simulink model "PMSM_FOC_CompVer"  (R2017b)
settings: Solver=FixedStepAuto  StartTime=0.0  StopTime=10.0  FixedStep=1e-6  RelTol=1e-3  AbsTol=1e-3
model workspace (MAT data in the model file):
  Ts = Simulink.Parameter
  Ts.Value = 0.001
  Ts.DataType = 'auto'
  Ts.Dimensions = [1 1]
libraries: nesl_utility x13, fl_lib x9, ee_lib x5, powerlib x4, simulink x3, powerlib_meascontrol x3, eeTransforms x2
settings Model: Creator=ljz  LastModifiedBy=ljz
settings DataIOCC: ReturnWorkspaceOutputs=on
settings DebuggingCC: SymbolicDimsDataTypeCodeGenerationDiagnostic=none
settings SFSimCC: SimUseLocalCustomCode=on
settings RTWCC: RTWUseLocalCustomCode=on
settings SimscapeCC: SimscapeLogType=all  SimscapeLogSimulationStatistics=on  SimscapeLogDataHistory=10000

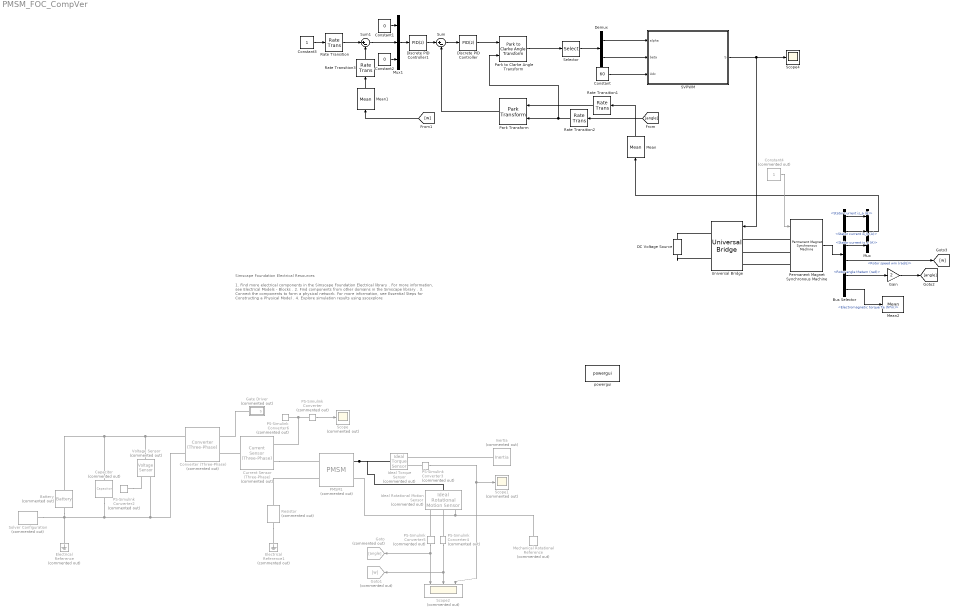
== system PMSM_FOC_CompVer ==
  note: 1. Find more electrical components in the Simscape Foundation Electrical library .
      | For more information, see Electrical Models - Blocks .
      | 2. Find components from other domains in the Simscape library .
      | 3. Connect the components to form a physical network.
      | For more information, see Essential Steps for Constructing a Physical Model .
      | 4. Explore simulation results using sscexplore
  note: Simscape Foundation Electrical Resources
  Battery : ee_lib/Sources/Battery  Commented=on  Vnom=12 V  R1=2 Ohm  prm_AH=1  AH=50 hr*A  V1=11.5 V  AH1=25 hr*A  prm_R2=1  R2=2000 Ohm  prm_dyn=1  Rp1=0.005 Ohm  tau1=30 s  Rp2=0.005 Ohm  tau2=30 s  Rp3=0.005 Ohm  tau3=30 s  Rp4=0.005 Ohm  tau4=30 s  Rp5=0.005 Ohm  tau5=30 s  prm_fade=1  N_fade=100  AH_fade=45 hr*A  R1_fade=2.02 Ohm  V1_fade=10.35 V  i_specify=off  i_priority=None  i=0 A  i_nominal_specify=off  i_nominal_unit=A  i_nominal_value=1  v_specify=off  v_priority=None  v=0 V  v_nominal_specify=off  v_nominal_unit=V  v_nominal_value=1  charge_specify=off  charge_priority=High  charge=50 hr*A  charge_nominal_specify=off  charge_nominal_unit=hr*A  charge_nominal_value=1  num_cycles_specify=off  num_cycles_priority=High  num_cycles=0  num_cycles_nominal_specify=off  num_cycles_nominal_unit=1  num_cycles_nominal_value=1  thermal_mass=30000 J/K  Tmeas=298.15 K  Vnom_T2=12 V  R1_T2=2.2 Ohm  V1_T2=11.4 V  R2_T2=2200 Ohm  Rp1_T2=0.005 Ohm  tau1_T2=30 s  Rp2_T2=0.005 Ohm  tau2_T2=30 s  Rp3_T2=0.005 Ohm  tau3_T2=30 s  Rp4_T2=0.005 Ohm  tau4_T2=30 s  Rp5_T2=0.005 Ohm  tau5_T2=30 s  Tmeas2=273.15 K  temperature_specify=off  temperature_priority=High  temperature=298.15 K  temperature_nominal_specify=off  temperature_nominal_unit=K  temperature_nominal_value=1
  Bus Selector : BusSelector  OutputSignals=Stator current is_a (A),Stator current is_b (A),Stator current is_c (A),Rotor speed wm (rad/s),Rotor angle thetam (rad),Electromagnetic torque Te (N*m)
  Capacitor : fl_lib/Electrical/Electrical Elements/Capacitor  Commented=on  c=220 uF  r=1e-6 Ohm  g=0 1/Ohm  i_specify=off  i_priority=None  i=0 A  i_nominal_specify=off  i_nominal_unit=A  i_nominal_value=1  v_specify=off  v_priority=None  v=0 V  v_nominal_specify=off  v_nominal_unit=V  v_nominal_value=1  vc_specify=off  vc_priority=High  vc=0 V  vc_nominal_specify=off  vc_nominal_unit=V  vc_nominal_value=1
  Constant : Constant  Value=60
  Constant1 : Constant  Value=0
  Constant2 : Constant  Value=0
  Constant3 : Constant
  Constant4 : Constant  Commented=on
  Converter (Three-Phase) : ee_lib/Semiconductors & Converters/Converters/Converter (Three-Phase)  Commented=on  device_type=ee.enum.converters.switchingdevice.ideal  Vf=0.8 V  Ron=0.001 Ohm  Rds=0.001 Ohm  Goff=1e-6 1/Ohm  Vth=0.5 V  Vgt=1 V  Vgt_off=-1 V  Ih=1 A  diode_param=ee.enum.converters.protectiondiode.none  diode_Vf=0.8 V  diode_Ron=0.001 Ohm  diode_Goff=1e-5 1/Ohm  diode_C=50 nF  diode_iRM=-235 A  diode_iF=300 A  diode_idot=-50 A/us  diode_trr_param=ee.enum.converters.diodetrr.trr_factor  diode_trr_factor=3  diode_trr=15 us  diode_Qrr=1500 s*uA  snubber_type=ee.enum.converters.snubber.exclude  Rs=0.1 Ohm  Cs=1e-7 F
      settings: SourceProductBaseCode=PS
  Current Sensor (Three-Phase) : ee_lib/Sensors & Transducers/Current Sensor (Three-Phase)  Commented=on
  DC Voltage Source : powerlib/Electrical Sources/DC Voltage Source  Amplitude=60  Measurements=None
  Demux : Demux  Outputs=2
  Discrete PID Controller : simulink/Continuous/PID Controller  Controller=PID  Form=Parallel  TimeDomain=Discrete-time  SampleTime=-1  IntegratorMethod=Forward Euler  FilterMethod=Forward Euler  ControllerParametersSource=internal  P=10  I=10  D=0  UseFilter=on  N=100  TunerSelectOption=Transfer Function Based (PID Tuner App)  InitialConditionSource=internal  InitialConditionForIntegrator=0  InitialConditionForFilter=0  DifferentiatorICPrevScaledInput=0  ExternalReset=none  TrackingMode=off  Kt=1  LimitOutput=off  UpperSaturationLimit=inf  LowerSaturationLimit=-inf  LinearizeAsGain=off  AntiWindupMode=none  Kb=1  POutMin=[]  POutMax=[]  IOutMin=[]  IOutMax=[]  DOutMin=[]  DOutMax=[]  NOutMin=[]  NOutMax=[]  SumOutMin=[]  SumOutMax=[]  SaturationOutMin=[]  SaturationOutMax=[]  PParamMin=[]  PParamMax=[]  IParamMin=[]  IParamMax=[]  DParamMin=[]  DParamMax=[]  NParamMin=[]  NParamMax=[]  KbParamMin=[]  KbParamMax=[]  KtParamMin=[]  KtParamMax=[]  KbOutMin=[]  KbOutMax=[]  KtOutMin=[]  KtOutMax=[]  IntegratorOutMin=[]  IntegratorOutMax=[]  FilterOutMin=[]  FilterOutMax=[]  SumI1OutMin=[]  SumI1OutMax=[]  SumI2OutMin=[]  SumI2OutMax=[]  SumI3OutMin=[]  SumI3OutMax=[]  SumDOutMin=[]  SumDOutMax=[]  DifferentiatorOutMin=[]  DifferentiatorOutMax=[]  FilterDiffOutCoefMin=[]  FilterDiffOutCoefMax=[]  ReciprocalOutMin=[]  ReciprocalOutMax=[]  SumDenOutMin=[]  SumDenOutMax=[]  SumNumOutMin=[]  SumNumOutMax=[]  DivideOutMin=[]  DivideOutMax=[]  IntegratorContinuousStateAttributes=''  IntegratorStateMustResolveToSignalObject=off  IntegratorRTWStateStorageClass=Auto  FilterContinuousStateAttributes=''  FilterStateMustResolveToSignalObject=off  FilterRTWStateStorageClass=Auto
  Discrete PID Controller1 : simulink/Continuous/PID Controller  Controller=PID  Form=Parallel  TimeDomain=Discrete-time  SampleTime=-1  IntegratorMethod=Forward Euler  FilterMethod=Forward Euler  ControllerParametersSource=internal  P=0.06  I=1  D=0  UseFilter=on  N=100  TunerSelectOption=Transfer Function Based (PID Tuner App)  InitialConditionSource=internal  InitialConditionForIntegrator=0  InitialConditionForFilter=0  DifferentiatorICPrevScaledInput=0  ExternalReset=none  TrackingMode=off  Kt=1  LimitOutput=off  UpperSaturationLimit=inf  LowerSaturationLimit=-inf  LinearizeAsGain=off  AntiWindupMode=none  Kb=1  POutMin=[]  POutMax=[]  IOutMin=[]  IOutMax=[]  DOutMin=[]  DOutMax=[]  NOutMin=[]  NOutMax=[]  SumOutMin=[]  SumOutMax=[]  SaturationOutMin=[]  SaturationOutMax=[]  PParamMin=[]  PParamMax=[]  IParamMin=[]  IParamMax=[]  DParamMin=[]  DParamMax=[]  NParamMin=[]  NParamMax=[]  KbParamMin=[]  KbParamMax=[]  KtParamMin=[]  KtParamMax=[]  KbOutMin=[]  KbOutMax=[]  KtOutMin=[]  KtOutMax=[]  IntegratorOutMin=[]  IntegratorOutMax=[]  FilterOutMin=[]  FilterOutMax=[]  SumI1OutMin=[]  SumI1OutMax=[]  SumI2OutMin=[]  SumI2OutMax=[]  SumI3OutMin=[]  SumI3OutMax=[]  SumDOutMin=[]  SumDOutMax=[]  DifferentiatorOutMin=[]  DifferentiatorOutMax=[]  FilterDiffOutCoefMin=[]  FilterDiffOutCoefMax=[]  ReciprocalOutMin=[]  ReciprocalOutMax=[]  SumDenOutMin=[]  SumDenOutMax=[]  SumNumOutMin=[]  SumNumOutMax=[]  DivideOutMin=[]  DivideOutMax=[]  IntegratorContinuousStateAttributes=''  IntegratorStateMustResolveToSignalObject=off  IntegratorRTWStateStorageClass=Auto  FilterContinuousStateAttributes=''  FilterStateMustResolveToSignalObject=off  FilterRTWStateStorageClass=Auto
  Electrical Reference : fl_lib/Electrical/Electrical Elements/Electrical Reference  Commented=on
  Electrical Reference1 : fl_lib/Electrical/Electrical Elements/Electrical Reference  Commented=on
  Gain : Gain  Gain=2
  Gate Driver : Subsystem  Commented=on
  Goto : Goto  Commented=on  GotoTag=angle
  Goto1 : Goto  Commented=on  GotoTag=w
  Ideal Rotational Motion Sensor : fl_lib/Mechanical/Mechanical Sensors/Ideal Rotational Motion Sensor  Commented=on  wrap_angle=simscape.enum.onoff.off  offset=0 rad
  Ideal Torque Sensor : fl_lib/Mechanical/Mechanical Sensors/Ideal Torque Sensor  Commented=on
  Inertia : fl_lib/Mechanical/Rotational Elements/Inertia  Commented=on  inertia=0.01 kg*m^2  w_specify=off  w_priority=High  w=0 rad/s  w_nominal_specify=off  w_nominal_unit=rad/s  w_nominal_value=1  t_specify=off  t_priority=None  t=0 N*m  t_nominal_specify=off  t_nominal_unit=N*m  t_nominal_value=1
  Mean : powerlib_meascontrol/Measurements/Mean  Freq=1000  Vinit=0  Ts=0
  Mean1 : powerlib_meascontrol/Measurements/Mean  Freq=1000  Vinit=0  Ts=0
  Mean2 : powerlib_meascontrol/Measurements/Mean  Freq=1000  Vinit=0  Ts=0
  Mechanical Rotational Reference : fl_lib/Mechanical/Rotational Elements/Mechanical Rotational Reference  Commented=on
  Mux : Mux  Inputs=3
  Mux1 : Mux  Inputs=3
  PMSM1 : ee_lib/Electromechanical/Permanent Magnet/PMSM  Commented=on  winding_type=ee.enum.statorconnection.wye  machine_param=ee.enum.pmsm.parameterization.constant  nPolePairs=6  pmflux_param=ee.enum.pmflux.fluxlinkage  pm_flux_linkage=0.03 Wb  torque_constant=0.18 N*m/A  back_emf_constant=0.18 V/(rad/s)  stator_param=ee.enum.statorparam.LdLqL0  Ld=0.00019 H  Lq=0.00025 H  idVec=[-200, 0, 200] A  iqVec=[-200, 0, 200] A  LdMatrix=0.0002 * ones(3, 3) H  LqMatrix=0.0002 * ones(3, 3) H  PmMatrix=0.1 * ones(3, 3) Wb  ktMatrix=0.18 * ones(3, 3) N*m/A  keMatrix=0.18 * ones(3, 3) V/(rad/s)  L0=0.00016 H  Ls=0.0002 H  Lm=-0.00002 H  Ms=0.00002 H  Rs=0.013 Ohm  zero_sequence=ee.enum.park.zerosequence.include  J=0.01 kg*m^2  lam=0 N*m/(rad/s)  axes_param=ee.enum.rotorangle.daxis  i_d_specify=off  i_d_priority=None  i_d=0 A  i_d_nominal_specify=off  i_d_nominal_unit=A  i_d_nominal_value=1  i_q_specify=off  i_q_priority=None  i_q=0 A  i_q_nominal_specify=off  i_q_nominal_unit=A  i_q_nominal_value=1  torque_specify=off  torque_priority=None  torque=0 N*m  torque_nominal_specify=off  torque_nominal_unit=N*m  torque_nominal_value=1  angular_velocity_specify=off  angular_velocity_priority=High  angular_velocity=0 rpm  angular_velocity_nominal_specify=off  angular_velocity_nominal_unit=rpm  angular_velocity_nominal_value=1  angular_position_specify=off  angular_position_priority=High  angular_position=0 deg  angular_position_nominal_specify=off  angular_position_nominal_unit=deg  angular_position_nominal_value=1  loss_param=ee.enum.ironloss.none  losses_oc=[0, 0, 0] W  losses_sc=[0, 0, 0] W  f_losses=60 Hz  Isc_losses=95 A  Tmeas=298.15 K  alpha=3.93e-3 1/K  alpha_flux=-0.001 1/K  stator_thermal_mass=100 J/K  rotor_thermal_mass=200 J/K  Rm_percent_rotor=90  Rd_percent_rotor=30  temperatureA_specify=off  temperatureA_priority=High  temperatureA=25 degC  temperatureA_nominal_specify=off  temperatureA_nominal_unit=degC  temperatureA_nominal_value=1  temperatureB_specify=off  temperatureB_priority=High  temperatureB=25 degC  temperatureB_nominal_specify=off  temperatureB_nominal_unit=degC  temperatureB_nominal_value=1  temperatureC_specify=off  temperatureC_priority=High  temperatureC=25 degC  temperatureC_nominal_specify=off  temperatureC_nominal_unit=degC  temperatureC_nominal_value=1  temperatureR_specify=off  temperatureR_priority=High  temperatureR=25 degC  temperatureR_nominal_specify=off  temperatureR_nominal_unit=degC  temperatureR_nominal_value=1
      settings: InternalSimscapePortConfiguration="{\"Bottom\":[],\"Left\":[{\"id\":\"N\",\"label\":\"~\",\"type\":\"foundation.electrical.three_phase\"},{\"id\":\"n\",\"label\":\"n\",\"type\":\"foundation.electrical.electrical\"}],\"Right\":[{\"id\":\"R\",\"label\":\"R\",\"type\":\"foundation.mechanical.rotational.rotational\"},{\"id\":\"C\",\"label\":\"C\",\"type\":\"foundation.mechanical.rotational.rotational\"}],\"Top\":[]}"
  PS-Simulink Converter{,2..6} (6 alike) : nesl_utility/PS-Simulink Converter  Commented=on  PhysicalDomain=network_engine_domain  SubClassName=ps_output  LeftPortType=input  RightPortType=output  PseudoPeriodic=off  Frequencies=[]  Unit=inherit  AffineConversion=off
  Park Transform : eeTransforms/Park Transform  AxisAlignment=D-axis  PowerInvariant=off
  Park to Clarke Angle Transform : eeTransforms/Park to Clarke Angle Transform  AxisAlignment=D-axis
      settings: SourceProductBaseCode=PS
  Permanent Magnet Synchronous Machine : powerlib/Machines/Permanent Magnet Synchronous Machine  NbPhases=3  FluxDistribution=Sinusoidal  RotorType=Round  MechanicalLoad=Torque Tm  PresetModel=No  ShowDetailedParameters=on  MeasurementBus=off  Resistance=18.7  Inductance=8.5e-3  dqInductances=[8.5e-3,8.5e-3]  La=0.02682  MachineConstant=Flux linkage established by magnets (V.s)  Flux=0.1716  VoltageCst=62.2496  TorqueCst=0.5148  Flat=120  Mechanical=[2.26e-05 1.349e-05 2 0]  PolePairs=2  InitialConditions=[0,0, 0,0]  InitialConditions5ph=[0 0 0 0 0 0]  RefAngle=Aligned with phase A axis (original Park)  IterativeDiscreteModel=Trapezoidal non iterative  TsBlock=-1  TsPowergui=0
  Rate Transition{,1..3} (4 alike) : RateTransition  OutPortSampleTime=0.001
  Resistor : fl_lib/Electrical/Electrical Elements/Resistor  Commented=on  R=100 Ohm  i_specify=off  i_priority=None  i=0 A  i_nominal_specify=off  i_nominal_unit=A  i_nominal_value=1  v_specify=off  v_priority=None  v=0 V  v_nominal_specify=off  v_nominal_unit=V  v_nominal_value=1
  SVPWM : Subsystem
  Scope : Scope  Commented=on
  Scope1 : Scope  Commented=on
  Scope2 : Scope  Commented=on  NumInputPorts=3
  Scope4 : Scope
  Selector : Selector  InputPortWidth=3  IndexOptions=Index vector (dialog)  Indices=[1 2]  OutputSizes=1
  Solver Configuration : nesl_utility/Solver Configuration  Commented=on  PhysicalDomain=network_engine_domain  SubClassName=solver  LeftPortType=input  RightPortType=generic  Tones=[]  Harmonics=[]  SimulateNoise=off  Profile=off  UseLocalSampling=off  EnableSwitchedLinearOptims=on  FrequencyDomain=off  UseCCode=off  RelTol=0.001  AbsTol=1e-06  MinStep=1e-09  ToWorkspace=off  RevertToSquareIcSolve=off  NumHomotopyIterations=100  PhasorMode=off  PhasorModeNumHarmonics=1  DoDC=off  ResidualTolerance=1e-09  UseLocalSolver=off  LocalSolverChoice=NE_BACKWARD_EULER_ADVANCER  LocalSolverSampleTime=0.001  DoFixedCost=off  MaxNonlinIter=3  MaxModeIter=2  LinearAlgebra=auto  EquationFormulation=NE_TIME_EF  DelaysMemoryBudget=1024  AutomaticFiltering=on  FilteringTimeConstant=0.001  PartitionStorageMethod=AS_NEEDED  PartitionMemoryBudget=1024  PartitionMethod=ROBUST
  Sum : Sum  Inputs=|+-
  Sum1 : Sum  Inputs=|+-
  Universal Bridge : powerlib/Power Electronics/Universal Bridge  Arms=3  SnubberResistance=1e5  SnubberCapacitance=inf  Device=IGBT / Diodes  Ron=1e-3  Lon=0  ForwardVoltages="[  0  0  ]"  ForwardVoltage=0  GTOparameters=[ 10e-6 , 20e-6 ]  IGBTparameters=[ 1e-6 , 2e-6 ]  Measurements=None  Measurements_2=None  converterType=Rectifier
  Voltage Sensor : fl_lib/Electrical/Electrical Sensors/Voltage Sensor  Commented=on
  powergui : powerlib/powergui  Priority=1  SimulationMode=Discrete  SampleTime=1e-6  frequency=60  Iterations=50  frequencyindice=0  Pbase=100e6  ErrMax=1e-4  UnitsV=kV  UnitsW=MW  buscounter=0  FunctionMessages=off  echomessages=off  EnableUseOfTLC=off  CurrentSourceSwitches=off  DisableSnubberDevices=off  DisableRonSwitches=off  DisableVfSwitches=off  DisplayEquations=off  AutomaticDiscreteSolvers=off  SolverType=Tustin/Backward Euler (TBE)  Interpol=off  ExternalGateDelay=off  methode=off  Ts=100  x0status=blocks  SPID=on  SwTol=0  HookPort=off  NonlinearTolerance=1e-4  nMaxIteration=100  ContinueOnMaxIteration=off  RestoreLinks=warning  ResistiveCurrentMeasurement=off  Frange=[0:2:500]  Ylog=off  Xlog=on  ShowGrid=off  save=off  variable=ZData  structure=0  ZoomFFT=off  StartTime=0.0  cycles=1  DisplayStyle=1  fundamental=60  FreqAxis=off  MaxFrequency=1000  frequencyindicesteady=1  RmsSteady=1  display=off
  wires:
  PS-Simulink Converter4/1 -> Goto1/1, Scope2/2
  PS-Simulink Converter3/1 -> Scope2/3, Scope1/1
  PS-Simulink Converter5/1 -> Scope2/1, Goto/1
  PS-Simulink Converter/1 -> Scope/1
  [angle] -> Rate Transition2/1
  Selector/1 -> Demux/1
  Park to Clarke Angle Transform/1 -> Selector/1
  Sum/1 -> Discrete PID Controller/1
  Discrete PID Controller/1 -> Park to Clarke Angle Transform/1
  Constant3/1 -> Rate Transition/1
  Rate Transition1/1 -> Park Transform/1
  Rate Transition2/1 -> Park to Clarke Angle Transform/2, Park Transform/2
  Permanent Magnet Synchronous Machine/1 -> Bus Selector/1
  Bus Selector/1 -> Mux/1  "<Stator current is_a (A)>"
  Bus Selector/2 -> Mux/2  "<Stator current is_b (A)>"
  Bus Selector/3 -> Mux/3  "<Stator current is_c (A)>"
  Mux/1 -> Mean/1
  Bus Selector/4 -> [w]  "<Rotor speed wm (rad/s)>"
  Bus Selector/5 -> Gain/1  "<Rotor angle thetam (rad)>"
  Park Transform/1 -> Sum/2
  Mean/1 -> Rate Transition1/1
  Gain/1 -> [angle]
  Demux/1 -> SVPWM/1(alpha)
  Demux/2 -> SVPWM/2(beta)
  Constant/1 -> SVPWM/3(Udc)
  SVPWM/1(S) -> Scope4/1, Universal Bridge/1
  Discrete PID Controller1/1 -> Sum/1
  [w] -> Mean1/1
  Mean1/1 -> Rate Transition3/1
  Rate Transition3/1 -> Sum1/2
  Rate Transition/1 -> Sum1/1
  Constant2/1 -> Mux1/3
  Constant1/1 -> Mux1/1
  Sum1/1 -> Mux1/2
  Mux1/1 -> Discrete PID Controller1/1
  Bus Selector/6 -> Mean2/1  "<Electromagnetic torque Te (N*m)>"
  Constant4/1 -> Permanent Magnet Synchronous Machine/1
  connections:
  Solver Configuration/RConn1 -- Battery/RConn1 -- Capacitor/RConn1 -- Voltage Sensor/RConn2 -- Converter (Three-Phase)/RConn2 -- Electrical Reference/LConn1
  PMSM1/RConn1 -- Ideal Rotational Motion Sensor/LConn1 -- Ideal Torque Sensor/LConn1
  Ideal Rotational Motion Sensor/RConn1 -- Mechanical Rotational Reference/LConn1 -- PMSM1/RConn2
  PS-Simulink Converter3/LConn1 -- Ideal Torque Sensor/RConn2
  Inertia/LConn1 -- Ideal Torque Sensor/RConn1
  PS-Simulink Converter4/LConn1 -- Ideal Rotational Motion Sensor/RConn2
  PS-Simulink Converter5/LConn1 -- Ideal Rotational Motion Sensor/RConn3
  Battery/LConn1 -- Capacitor/LConn1 -- Voltage Sensor/LConn1 -- Converter (Three-Phase)/RConn1
  PS-Simulink Converter2/LConn1 -- Voltage Sensor/RConn1
  Gate Driver/RConn1 -- Converter (Three-Phase)/LConn1
  Current Sensor (Three-Phase)/LConn1 -- Converter (Three-Phase)/LConn2
  Current Sensor (Three-Phase)/RConn2 -- PMSM1/LConn1
  PS-Simulink Converter/LConn1 -- PS-Simulink Converter6/LConn1 -- Current Sensor (Three-Phase)/RConn1
  PMSM1/LConn2 -- Resistor/LConn1
  Resistor/RConn1 -- Electrical Reference1/LConn1
  Permanent Magnet Synchronous Machine/LConn1 -- Universal Bridge/LConn1
  Permanent Magnet Synchronous Machine/LConn2 -- Universal Bridge/LConn2
  Permanent Magnet Synchronous Machine/LConn3 -- Universal Bridge/LConn3
  DC Voltage Source/RConn1 -- Universal Bridge/RConn1
  DC Voltage Source/LConn1 -- Universal Bridge/RConn2

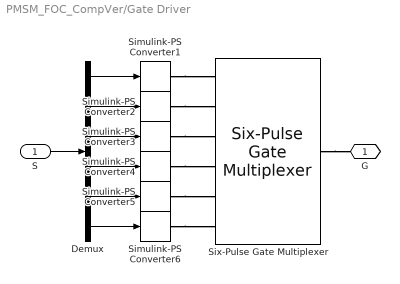
== system PMSM_FOC_CompVer/Gate Driver ==
  S : Inport
  Demux : Demux  Outputs=6
  Simulink-PS Converter{1..6} (6 alike) : nesl_utility/Simulink-PS Converter  PhysicalDomain=network_engine_domain  SubClassName=ps_input  LeftPortType=input  RightPortType=output  PseudoPeriodic=off  Frequencies=[]  NoiseDistribution=none  NoiseParameters=[]  Unit=1  AffineConversion=off  FilteringAndDerivatives=zero  SimscapeFilterOrder=1  InputFilterTimeConstant=0.001  UdotUserProvided=1
  Six-Pulse Gate Multiplexer : ee_lib/Semiconductors & Converters/Converters/Six-Pulse Gate Multiplexer  R=0 Ohm
      settings: SourceProductBaseCode=PS  InternalSimscapePortConfiguration="{\"Bottom\":[],\"Left\":[{\"id\":\"GaH\",\"label\":\"Ga(H)\",\"type\":\"input\"},{\"id\":\"GaL\",\"label\":\"Ga(L)\",\"type\":\"input\"},{\"id\":\"GbH\",\"label\":\"Gb(H)\",\"type\":\"input\"},{\"id\":\"GbL\",\"label\":\"Gb(L)\",\"type\":\"input\"},{\"id\":\"GcH\",\"label\":\"Gc(H)\",\"type\":\"input\"},{\"id\":\"GcL\",\"label\":\"Gc(L)\",\"type\":\"input\"}],\"Right\":[{\"id\":\"p\",\"label\":\"G\",\"type\":\"foundation.electrical.twelve_phase\"}],\"Top\":[]}"
  G : PMIOPort  Side=Right
  wires:
  Demux/1 -> Simulink-PS Converter1/1
  S/1 -> Demux/1
  Demux/4 -> Simulink-PS Converter4/1
  Demux/2 -> Simulink-PS Converter2/1
  Demux/3 -> Simulink-PS Converter3/1
  Demux/5 -> Simulink-PS Converter5/1
  Demux/6 -> Simulink-PS Converter6/1
  connections:
  Six-Pulse Gate Multiplexer/RConn1 -- G/RConn1
  Simulink-PS Converter1/RConn1 -- Six-Pulse Gate Multiplexer/LConn1
  Simulink-PS Converter3/RConn1 -- Six-Pulse Gate Multiplexer/LConn3
  Simulink-PS Converter5/RConn1 -- Six-Pulse Gate Multiplexer/LConn5
  Simulink-PS Converter6/RConn1 -- Six-Pulse Gate Multiplexer/LConn6
  Simulink-PS Converter4/RConn1 -- Six-Pulse Gate Multiplexer/LConn4
  Simulink-PS Converter2/RConn1 -- Six-Pulse Gate Multiplexer/LConn2

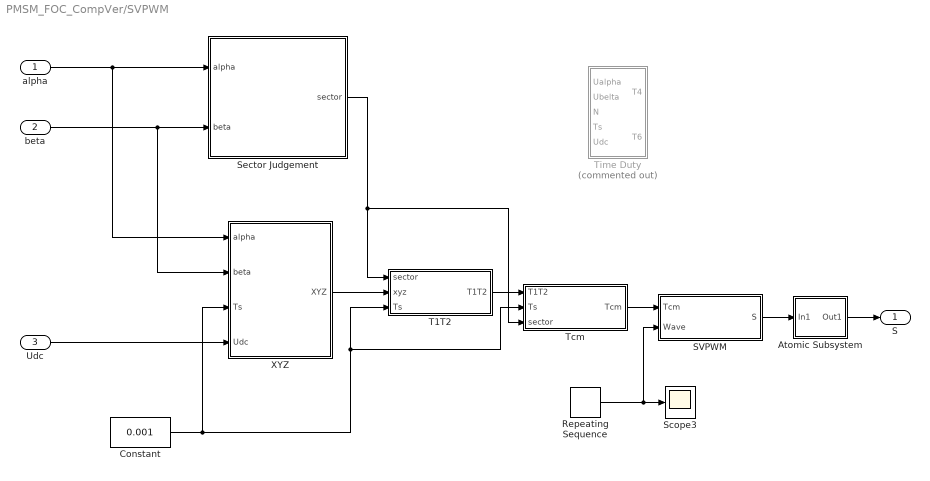
== system PMSM_FOC_CompVer/SVPWM ==
  alpha : Inport
  beta : Inport  Port=2
  Udc : Inport  Port=3
  Atomic Subsystem : Subsystem  TreatAsAtomicUnit=on
  Constant : Constant  Value=0.001
  Repeating Sequence : simulink/Sources/Repeating Sequence  rep_seq_t=[0 Ts/2 Ts]  rep_seq_y=[0 Ts 0]
  SVPWM : Subsystem  TreatAsAtomicUnit=on
  Scope3 : Scope
  Sector Judgement : Subsystem  TreatAsAtomicUnit=on
  T1T2 : Subsystem  TreatAsAtomicUnit=on
  Tcm : Subsystem  TreatAsAtomicUnit=on
  Time Duty : Subsystem  Commented=on
  XYZ : Subsystem  TreatAsAtomicUnit=on
  S : Outport
  wires:
  beta/1 -> XYZ/2(beta), Sector Judgement/2(beta)
  Sector Judgement/1(sector) -> T1T2/1(sector), Tcm/3(sector)
  alpha/1 -> XYZ/1(alpha), Sector Judgement/1(alpha)
  Tcm/1(Tcm) -> SVPWM/1(Tcm)
  Repeating Sequence/1 -> Scope3/1, SVPWM/2(Wave)
  Constant/1 -> XYZ/3(Ts), Tcm/2(Ts), T1T2/3(Ts)
  SVPWM/1(S) -> Atomic Subsystem/1(In1)
  XYZ/1(XYZ) -> T1T2/2(xyz)
  T1T2/1(T1T2) -> Tcm/1(T1T2)
  Udc/1 -> XYZ/4(Udc)
  Atomic Subsystem/1(Out1) -> S/1

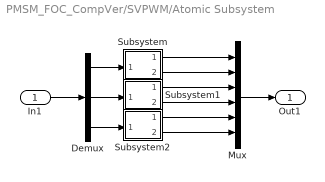
== system PMSM_FOC_CompVer/SVPWM/Atomic Subsystem ==
  In1 : Inport
  Demux : Demux  Outputs=3
  Mux : Mux  Inputs=6
  Subsystem : Subsystem
  Subsystem1 : Subsystem
  Subsystem2 : Subsystem
  Out1 : Outport
  wires:
  Demux/2 -> Subsystem1/1(In1)
  In1/1 -> Demux/1
  Demux/1 -> Subsystem/1(In1)
  Demux/3 -> Subsystem2/1(In1)
  Subsystem/2(Out2) -> Mux/2
  Subsystem1/2(Out2) -> Mux/4
  Subsystem2/2(Out2) -> Mux/6
  Subsystem/1(Out1) -> Mux/1
  Subsystem1/1(Out1) -> Mux/3
  Subsystem2/1(Out1) -> Mux/5
  Mux/1 -> Out1/1

== system PMSM_FOC_CompVer/SVPWM/SVPWM ==
  Tcm : Inport
  Wave : Inport  Port=2
  Add : Sum  Inputs=+-
  Constant : Constant  Value=0
  Constant1 : Constant
  Switch : Switch  Criteria=u2 > Threshold
  S : Outport
  wires:
  Tcm/1 -> Add/1
  Wave/1 -> Add/2
  Add/1 -> Switch/2
  Constant/1 -> Switch/1
  Constant1/1 -> Switch/3
  Switch/1 -> S/1

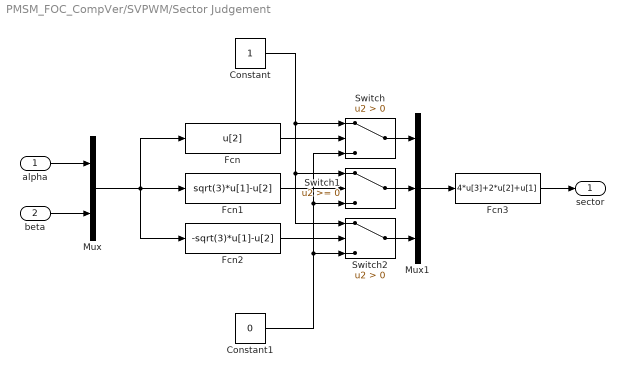
== system PMSM_FOC_CompVer/SVPWM/Sector Judgement ==
  alpha : Inport
  beta : Inport  Port=2
  Constant : Constant
  Constant1 : Constant  Value=0
  Fcn : Fcn  Expr=u[2]
  Fcn1 : Fcn  Expr=sqrt(3)*u[1]-u[2]
  Fcn2 : Fcn  Expr=-sqrt(3)*u[1]-u[2]
  Fcn3 : Fcn  Expr=4*u[3]+2*u[2]+u[1]
  Mux : Mux  Inputs=2
  Mux1 : Mux  Inputs=3
  Switch : Switch  Criteria=u2 > Threshold
  Switch1 : Switch
  Switch2 : Switch  Criteria=u2 > Threshold
  sector : Outport
  wires:
  alpha/1 -> Mux/1
  beta/1 -> Mux/2
  Mux/1 -> Fcn1/1, Fcn2/1, Fcn/1
  Fcn/1 -> Switch/2
  Fcn1/1 -> Switch1/2
  Fcn2/1 -> Switch2/2
  Constant1/1 -> Switch2/3, Switch1/3, Switch/3
  Constant/1 -> Switch2/1, Switch1/1, Switch/1
  Switch2/1 -> Mux1/3
  Switch/1 -> Mux1/1
  Switch1/1 -> Mux1/2
  Mux1/1 -> Fcn3/1
  Fcn3/1 -> sector/1

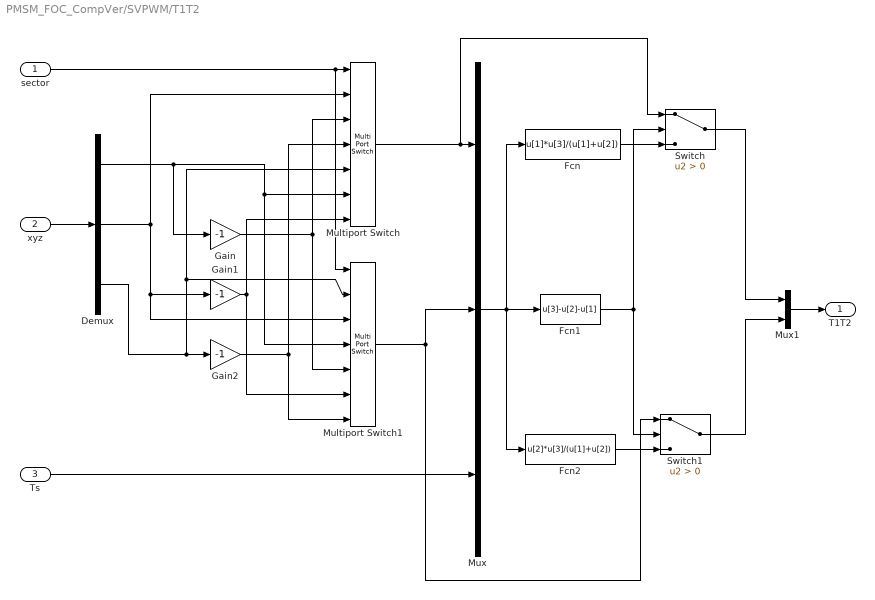
== system PMSM_FOC_CompVer/SVPWM/T1T2 ==
  sector : Inport
  xyz : Inport  Port=2
  Ts : Inport  Port=3
  Demux : Demux  Outputs=3
  Fcn : Fcn  Expr=u[1]*u[3]/(u[1]+u[2])
  Fcn1 : Fcn  Expr=u[3]-u[2]-u[1]
  Fcn2 : Fcn  Expr=u[2]*u[3]/(u[1]+u[2])
  Gain : Gain  Gain=-1
  Gain1 : Gain  Gain=-1
  Gain2 : Gain  Gain=-1
  Multiport Switch : MultiPortSwitch  Inputs=6
  Multiport Switch1 : MultiPortSwitch  Inputs=6
  Mux : Mux  Inputs=3
  Mux1 : Mux  Inputs=2
  Switch : Switch  Criteria=u2 > Threshold
  Switch1 : Switch  Criteria=u2 > Threshold
  T1T2 : Outport
  wires:
  xyz/1 -> Demux/1
  Demux/1 -> Multiport Switch/6, Multiport Switch1/4, Gain/1
  Demux/2 -> Multiport Switch/2, Gain1/1, Multiport Switch1/3
  Demux/3 -> Gain2/1, Multiport Switch1/2, Multiport Switch/5
  sector/1 -> Multiport Switch1/1, Multiport Switch/1
  Multiport Switch/1 -> Switch/1, Mux/1
  Multiport Switch1/1 -> Switch1/1, Mux/2
  Ts/1 -> Mux/3
  Mux/1 -> Fcn2/1, Fcn/1, Fcn1/1
  Fcn1/1 -> Switch1/2, Switch/2
  Mux1/1 -> T1T2/1
  Switch/1 -> Mux1/1
  Switch1/1 -> Mux1/2
  Fcn/1 -> Switch/3
  Fcn2/1 -> Switch1/3
  Gain2/1 -> Multiport Switch1/7, Multiport Switch/4
  Gain/1 -> Multiport Switch/3, Multiport Switch1/5
  Gain1/1 -> Multiport Switch1/6, Multiport Switch/7

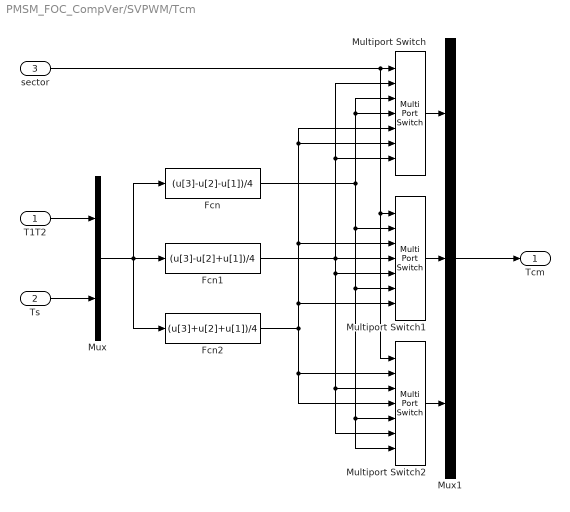
== system PMSM_FOC_CompVer/SVPWM/Tcm ==
  T1T2 : Inport
  Ts : Inport  Port=2
  sector : Inport  Port=3
  Fcn : Fcn  Expr=(u[3]-u[2]-u[1])/4
  Fcn1 : Fcn  Expr=(u[3]-u[2]+u[1])/4
  Fcn2 : Fcn  Expr=(u[3]+u[2]+u[1])/4
  Multiport Switch : MultiPortSwitch  Inputs=6
  Multiport Switch1 : MultiPortSwitch  Inputs=6
  Multiport Switch2 : MultiPortSwitch  Inputs=6
  Mux : Mux  Inputs=2
  Mux1 : Mux  Inputs=3
  Tcm : Outport
  wires:
  T1T2/1 -> Mux/1
  Ts/1 -> Mux/2
  Mux/1 -> Fcn2/1, Fcn1/1, Fcn/1
  Fcn/1 -> Multiport Switch1/2, Multiport Switch2/5, Multiport Switch2/7, Multiport Switch1/6, Multiport Switch/3, Multiport Switch/4
  Fcn1/1 -> Multiport Switch1/4, Multiport Switch2/6, Multiport Switch2/3, Multiport Switch1/5, Multiport Switch/7, Multiport Switch/2
  Fcn2/1 -> Multiport Switch2/2, Multiport Switch2/4, Multiport Switch1/7, Multiport Switch1/3, Multiport Switch/5, Multiport Switch/6
  sector/1 -> Multiport Switch2/1, Multiport Switch1/1, Multiport Switch/1
  Multiport Switch/1 -> Mux1/1
  Multiport Switch1/1 -> Mux1/2
  Multiport Switch2/1 -> Mux1/3
  Mux1/1 -> Tcm/1

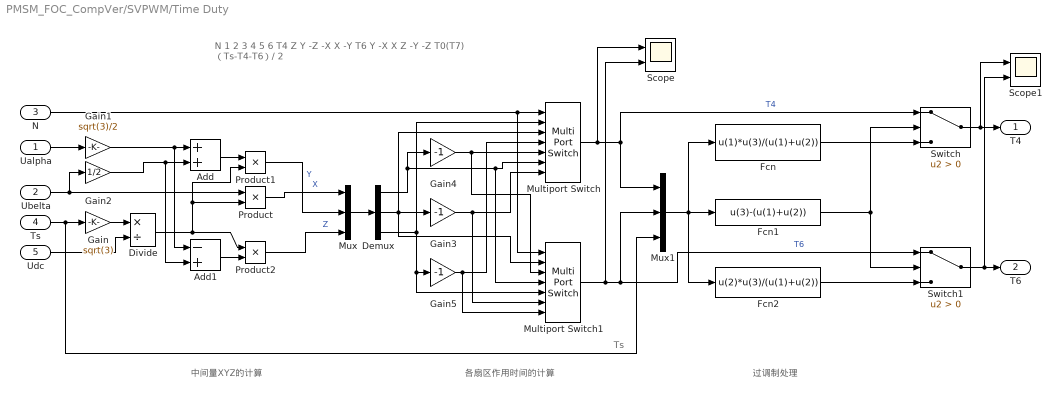
== system PMSM_FOC_CompVer/SVPWM/Time Duty ==
  note: N		1		2		3		4		5		6
      | T4		Z		Y		-Z		-X		X		-Y
      | T6		Y		-X		X		Z		-Y		-Z
      | T0(T7)		（Ts-T4-T6）/ 2
  note: 过调制处理
  note: 中间量XYZ的计算
  note: Ts
  note: 各扇区作用时间的计算
  Ualpha : Inport
  Ubelta : Inport  Port=2
  N : Inport  Port=3
  Ts : Inport  Port=4
  Udc : Inport  Port=5
  Add : Sum
  Add1 : Sum  Inputs=-+
  Demux : Demux  Outputs=3
  Divide : Product  Inputs=*/
  Fcn : Fcn  Expr=u(1)*u(3)/(u(1)+u(2))
  Fcn1 : Fcn  Expr=u(3)-(u(1)+u(2))
  Fcn2 : Fcn  Expr=u(2)*u(3)/(u(1)+u(2))
  Gain : Gain  Gain=sqrt(3)
  Gain1 : Gain  Gain=sqrt(3)/2
  Gain2 : Gain  Gain=1/2
  Gain3 : Gain  Gain=-1
  Gain4 : Gain  Gain=-1
  Gain5 : Gain  Gain=-1
  Multiport Switch : MultiPortSwitch  DataPortOrder=Specify indices  Inputs=6  DataPortIndices={1,2,3,4,5,6}
  Multiport Switch1 : MultiPortSwitch  DataPortOrder=Specify indices  Inputs=6  DataPortIndices={1,2,3,4,5,6}
  Mux : Mux  Inputs=3
  Mux1 : Mux  Inputs=3
  Product : Product
  Product1 : Product
  Product2 : Product
  Scope : Scope  NumInputPorts=2
  Scope1 : Scope  NumInputPorts=2
  Switch : Switch  Criteria=u2 > Threshold
  Switch1 : Switch  Criteria=u2 > Threshold
  T4 : Outport
  T6 : Outport  Port=2
  wires:
  Gain2/1 -> Add1/2, Add/2
  Add/1 -> Product1/1
  Ubelta/1 -> Product/1, Gain2/1
  Gain1/1 -> Add1/1, Add/1
  Udc/1 -> Divide/2
  Add1/1 -> Product2/2
  Ts/1 -> Mux1/3, Gain/1
  Gain/1 -> Divide/1
  Divide/1 -> Product1/2, Product/2, Product2/1
  Ualpha/1 -> Gain1/1
  Product1/1 -> Mux/2  "Y"
  N/1 -> Multiport Switch1/1, Multiport Switch/1
  Mux/1 -> Demux/1
  Demux/3 -> Gain5/1, Multiport Switch1/5, Multiport Switch/2
  Demux/2 -> Multiport Switch1/2, Multiport Switch/3, Gain3/1
  Gain5/1 -> Multiport Switch1/7, Multiport Switch/4
  Demux/1 -> Gain4/1, Multiport Switch1/4, Multiport Switch/6
  Gain4/1 -> Multiport Switch1/3, Multiport Switch/5
  Gain3/1 -> Multiport Switch1/6, Multiport Switch/7
  Multiport Switch/1 -> Scope/1, Switch/1, Mux1/1  "T4"
  Multiport Switch1/1 -> Scope/2, Switch1/1, Mux1/2  "T6"
  Mux1/1 -> Fcn2/1, Fcn/1, Fcn1/1
  Fcn/1 -> Switch/3
  Fcn1/1 -> Switch/2, Switch1/2
  Fcn2/1 -> Switch1/3
  Switch/1 -> Scope1/1, T4/1
  Switch1/1 -> Scope1/2, T6/1
  Product2/1 -> Mux/3  "Z"
  Product/1 -> Mux/1  "X"

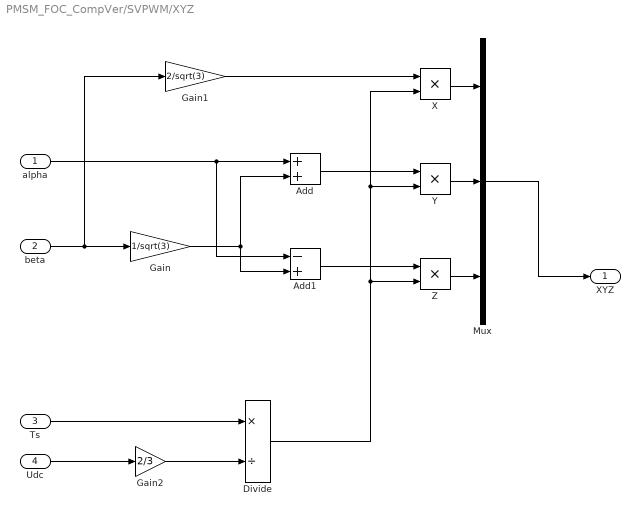
== system PMSM_FOC_CompVer/SVPWM/XYZ ==
  alpha : Inport
  beta : Inport  Port=2
  Ts : Inport  Port=3
  Udc : Inport  Port=4
  Add : Sum
  Add1 : Sum  Inputs=-+
  Divide : Product  Inputs=*/
  Gain : Gain  Gain=1/sqrt(3)
  Gain1 : Gain  Gain=2/sqrt(3)
  Gain2 : Gain  Gain=2/3
  Mux : Mux  Inputs=3
  X : Product  Inputs=**
  Y : Product  Inputs=**
  Z : Product  Inputs=**
  XYZ : Outport
  wires:
  beta/1 -> Gain/1, Gain1/1
  alpha/1 -> Add/1, Add1/1
  Gain/1 -> Add1/2, Add/2
  Ts/1 -> Divide/1
  Udc/1 -> Gain2/1
  Gain2/1 -> Divide/2
  Add/1 -> Y/1
  Add1/1 -> Z/1
  Gain1/1 -> X/1
  Divide/1 -> X/2, Y/2, Z/2
  X/1 -> Mux/1
  Y/1 -> Mux/2
  Z/1 -> Mux/3
  Mux/1 -> XYZ/1

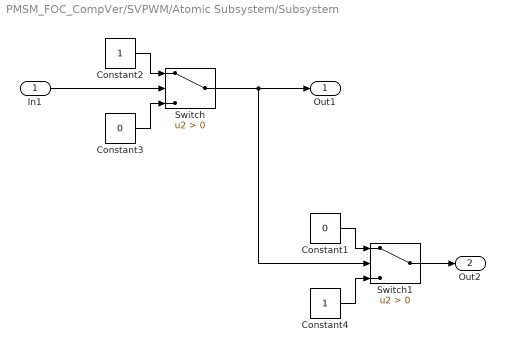
== system PMSM_FOC_CompVer/SVPWM/Atomic Subsystem/Subsystem ==
  In1 : Inport
  Constant1 : Constant  Value=0
  Constant2 : Constant
  Constant3 : Constant  Value=0
  Constant4 : Constant
  Switch : Switch  Criteria=u2 > Threshold
  Switch1 : Switch  Criteria=u2 > Threshold
  Out1 : Outport
  Out2 : Outport  Port=2
  wires:
  Constant2/1 -> Switch/1
  Switch1/1 -> Out2/1
  Constant3/1 -> Switch/3
  In1/1 -> Switch/2
  Switch/1 -> Switch1/2, Out1/1
  Constant1/1 -> Switch1/1
  Constant4/1 -> Switch1/3

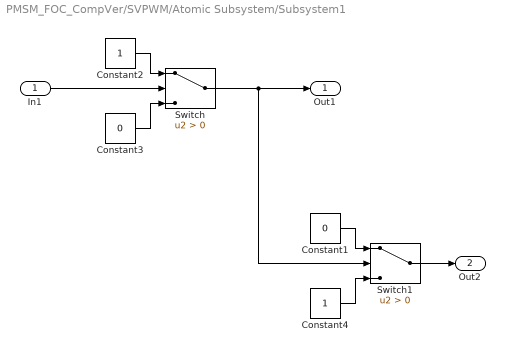
== system PMSM_FOC_CompVer/SVPWM/Atomic Subsystem/Subsystem1 ==
  In1 : Inport
  Constant1 : Constant  Value=0
  Constant2 : Constant
  Constant3 : Constant  Value=0
  Constant4 : Constant
  Switch : Switch  Criteria=u2 > Threshold
  Switch1 : Switch  Criteria=u2 > Threshold
  Out1 : Outport
  Out2 : Outport  Port=2
  wires:
  Constant2/1 -> Switch/1
  Switch1/1 -> Out2/1
  Constant3/1 -> Switch/3
  In1/1 -> Switch/2
  Switch/1 -> Switch1/2, Out1/1
  Constant1/1 -> Switch1/1
  Constant4/1 -> Switch1/3

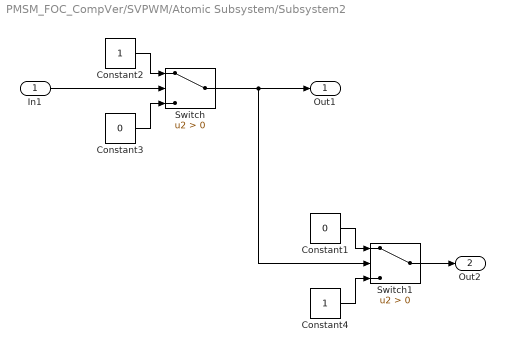
== system PMSM_FOC_CompVer/SVPWM/Atomic Subsystem/Subsystem2 ==
  In1 : Inport
  Constant1 : Constant  Value=0
  Constant2 : Constant
  Constant3 : Constant  Value=0
  Constant4 : Constant
  Switch : Switch  Criteria=u2 > Threshold
  Switch1 : Switch  Criteria=u2 > Threshold
  Out1 : Outport
  Out2 : Outport  Port=2
  wires:
  Constant2/1 -> Switch/1
  Switch1/1 -> Out2/1
  Constant3/1 -> Switch/3
  In1/1 -> Switch/2
  Switch/1 -> Switch1/2, Out1/1
  Constant1/1 -> Switch1/1
  Constant4/1 -> Switch1/3
